simulink model "LQR_model_output_observer"  (R2019a)
settings: Solver=FixedStepAuto  StartTime=0.0  StopTime=inf  FixedStep=Ts  RelTol=1e-3  EnableMultiTasking=on
values from neighbouring files (symbols this model uses):
  K_lqr = [-70.7107 -83.3587 -91.2872 -13.2266]    [LQR_params.m]
  max_velocity =     [LQR_params.m]
  p_ref = 0    [LQR_params.m]
  theta_ref =     [LQR_params.m]
libraries: simulink x2
settings Model: SimulationMode=external  Creator=rahelrickenbach  LastModifiedBy=christinefux
settings SolverCC: PositivePriorityOrder=on
settings OptimizationCC: EnhancedBackFolding=on  PassReuseOutputArgsAs=Individual arguments  MaxStackSize=64  OptimizeBlockOrder=speed  DifferentSizesBufferReuse=on  OptimizationCustomize=off
settings DebuggingCC: ParameterTunabilityLossMsg=error
settings HardwareCC: ProdBitPerPointer=32  ProdBitPerSizeT=32  ProdBitPerPtrDiffT=32  ProdLargestAtomicInteger=Long  ProdLargestAtomicFloat=Double  ProdWordSize=32  ProdLongLongMode=on  ProdHWDeviceType=ARM Compatible->ARM Cortex
settings SFSimCC: MATLABDynamicMemAlloc=off
settings RTWCC: SystemTargetFile=ert.tlc  HardwareBoard=Raspberry Pi  TLCOptions="-aInlineSetEventsForThisBaseRateFcn=TLC_FALSE -aSuppressMultiTaskScheduler=TLC_FALSE  -aRateBasedStepFcn=0"  TemplateMakefile=ert_default_tmf  GenerateReport=on  Toolchain=GNU GCC Raspberry Pi  IncludeHyperlinkInReport=on  LaunchReport=on  GenerateTraceInfo=on  GenerateTraceReport=on  GenerateTraceReportSl=on  GenerateTraceReportSf=on  GenerateTraceReportEml=on
settings CodeAppCC: ForceParamTrailComments=on  IgnoreCustomStorageClasses=off  MaxIdLength=63  OperatorAnnotations=on  SimulinkDataObjDesc=on  SFDataObjDesc=on  InsertBlockDesc=on
settings ERTTargetCC: SupportVariableSizeSignals=on

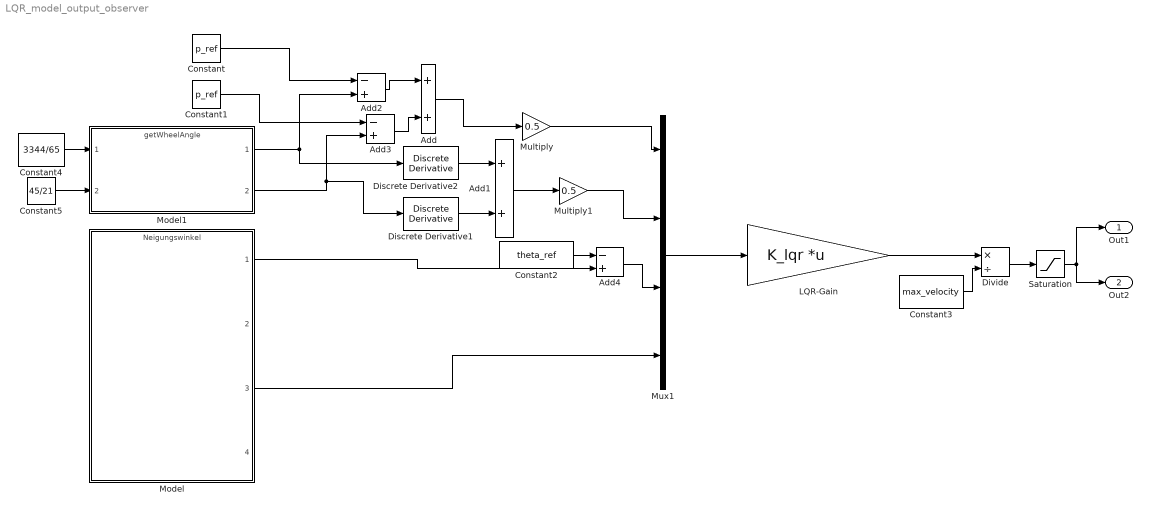
== system LQR_model_output_observer ==
  Add : Sum
  Add1 : Sum
  Add2 : Sum  Inputs=-+
  Add3 : Sum  Inputs=-+
  Add4 : Sum  Inputs=-+
  Constant : Constant  Value=p_ref  OutDataTypeStr=single
  Constant1 : Constant  Value=p_ref  OutDataTypeStr=single
  Constant2 : Constant  Value=theta_ref  OutDataTypeStr=single
  Constant3 : Constant  Value=max_velocity  OutDataTypeStr=single
  Constant4 : Constant  Value=3344/65
  Constant5 : Constant  Value=45/21
  Discrete Derivative1 : simulink/Discrete/Discrete Derivative  gainval=1.0  ICPrevScaledInput=0.0  OutMin=[]  OutMax=[]  OutDataType=fixdt(1, 16)  OutScaling=2^-10  DoSatur=off
  Discrete Derivative2 : simulink/Discrete/Discrete Derivative  gainval=1.0  ICPrevScaledInput=0.0  OutMin=[]  OutMax=[]  OutDataType=fixdt(1, 16)  OutScaling=2^-10  DoSatur=off
  Divide : Product  Inputs=*/
  LQR-Gain : Gain  Gain=K_lqr  Multiplication=Matrix(K*u) (u vector)
  Model : ModelReference  ModelNameDialog=Neigungswinkel  SimulationMode=Normal  ModelReferenceVersion=1.60
  Model1 : ModelReference  ModelNameDialog=getWheelAngle.slx  SimulationMode=Normal  ModelReferenceVersion=1.23
  Multiply : Gain  Gain=0.5
  Multiply1 : Gain  Gain=0.5
  Mux1 : Mux
  Saturation : Saturate  UpperLimit=1  LowerLimit=-1
  Out1 : Outport
  Out2 : Outport  Port=2
  wires:
  Model1/1 -> Add2/2, Discrete Derivative2/1
  Model1/2 -> Discrete Derivative1/1, Add3/2
  Add/1 -> Multiply/1
  Discrete Derivative2/1 -> Add1/1
  Discrete Derivative1/1 -> Add1/2
  Add1/1 -> Multiply1/1
  Multiply1/1 -> Mux1/2
  Constant/1 -> Add2/1
  Add2/1 -> Add/1
  Constant1/1 -> Add3/1
  Add3/1 -> Add/2
  Constant2/1 -> Add4/1
  Add4/1 -> Mux1/3
  Constant3/1 -> Divide/2
  Divide/1 -> Saturation/1
  Saturation/1 -> Out2/1, Out1/1
  Constant4/1 -> Model1/1
  Constant5/1 -> Model1/2
  Model/1 -> Add4/2
  Mux1/1 -> LQR-Gain/1
  LQR-Gain/1 -> Divide/1
  Model/3 -> Mux1/4
  Multiply/1 -> Mux1/1
